simulink model "Simulink_test_tiberlot"  (R2015a)
settings: Solver=ode45  StartTime=0.0  StopTime=10.0  RelTol=1e-3
values from neighbouring files (symbols this model uses):
  intervalle_tau = [1 12]    [Savitsky1964_statique_input_power.m]    (also in Savitsky1964_statique_input_power_old.m; test_tiberlot.m)
  vx = 22    [test_tiberlot.m]
settings Model: Creator=charl  LastModifiedBy=charl

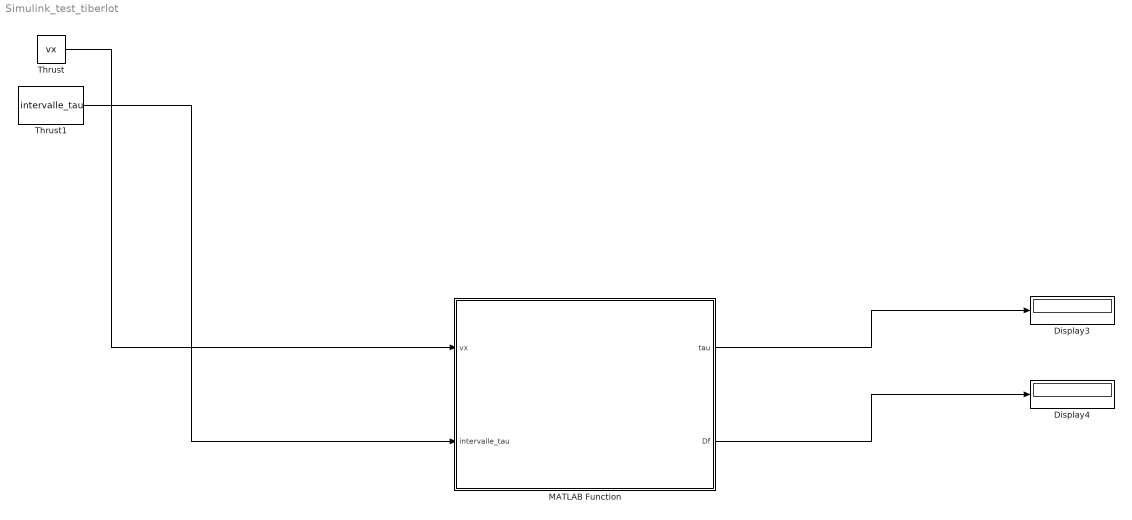
== system Simulink_test_tiberlot ==
  Display3 : Display
  Display4 : Display
  MATLAB Function : MATLAB Function  TreatAsAtomicUnit=on
  Thrust : Constant  Value=vx
  Thrust1 : Constant  Value=intervalle_tau
  wires:
  Thrust/1 -> MATLAB Function/1(vx)
  Thrust1/1 -> MATLAB Function/2(intervalle_tau)
  MATLAB Function/1(tau) -> Display3/1
  MATLAB Function/2(Df) -> Display4/1

== matlab function Simulink_test_tiberlot/MATLAB Function ==
  data: vx input size=1; tau output size=1; intervalle_tau input size=2; Df output size=1; SimulinkParam parameter
function [tau,Df] = Call_Savitsky1964_statique_input_vitesse_fcn(vx,intervalle_tau, SimulinkParam)
% fonction pour caller Savitsky1964_statique_input_vitesse_fcn
% global g
% global rho
% global m L LCG VCG b beta a f epsilon
coder.extrinsic('Savitsky1964_statique_input_vitesse_fcn');

tau = 0;Df=0;
CstData  = SimulinkParam;
% CstData = 0 ;
[tau,~,~,Df] = Savitsky1964_statique_input_vitesse_fcn(vx,intervalle_tau,CstData);
%%
%% Ajouter les variables globales
% GlobalHullGeometry('SavitskyExample'); % load hull geometry
% GlobalHullGeometry('Cedarville');
% global m L LCG VCG b beta a f epsilon
% global g
% g = 9.81;% m/s2, accélération gravitationnelle
% global rho
% rho = 1000; % kg/m3; eau douce = 1000; eau salée = 1025
% Planing coefficients
% Cv = v/sqrt(g*b);
% CL_beta = m*g/(0.5*rho*v^2*b^2);% lift coefficient pour un angle beta.
% Déjà calculés dans la fonction statique_input_vitesse_v2
% Calculs
% [tau, ~,Df] = bissection_fcn_v_input(intervalle_tau(1),intervalle_tau(end),0.001,vx);
% P_e = D_e*v;
